simulink model "sxqq08022311"  (R2022b)
settings: Solver=VariableStepAuto  StartTime=0.0  StopTime=0.2  RelTol=1e-3
libraries: spsVoltageMeasurementLib x14, spsThyristorLib x6, spsCurrentMeasurementLib x3, spsACVoltageSourceLib x3, spsSeriesRLCBranchLib x2, spsGroundLib x1, powerlib_extras x1, spsUniversalBridgeLib x1, sps_lib x1
settings Model: Creator=赵晨琨  LastModifiedBy=ASUS
settings SolverCC: AlgebraicLoopSolver=TrustRegion
settings DataIOCC: Refine=3
settings DebuggingCC: UnconnectedInputMsg=warning  UnconnectedOutputMsg=warning  UnconnectedLineMsg=warning  SFMachineParentedDataDiag=warning
settings ModelReferenceCC: EnableRefExpFcnMdlSchedulingChecks=on

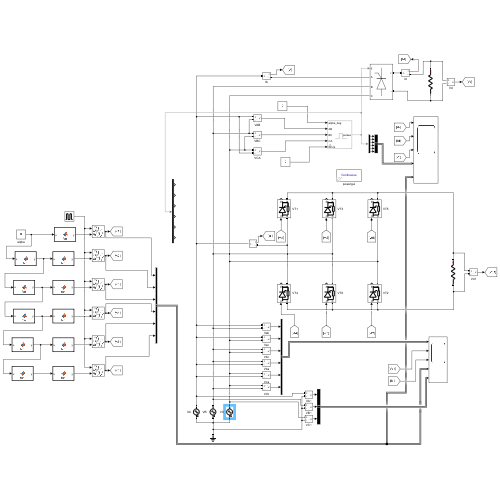
[thumbnail: Simulink's stored preview of the top-level diagram]
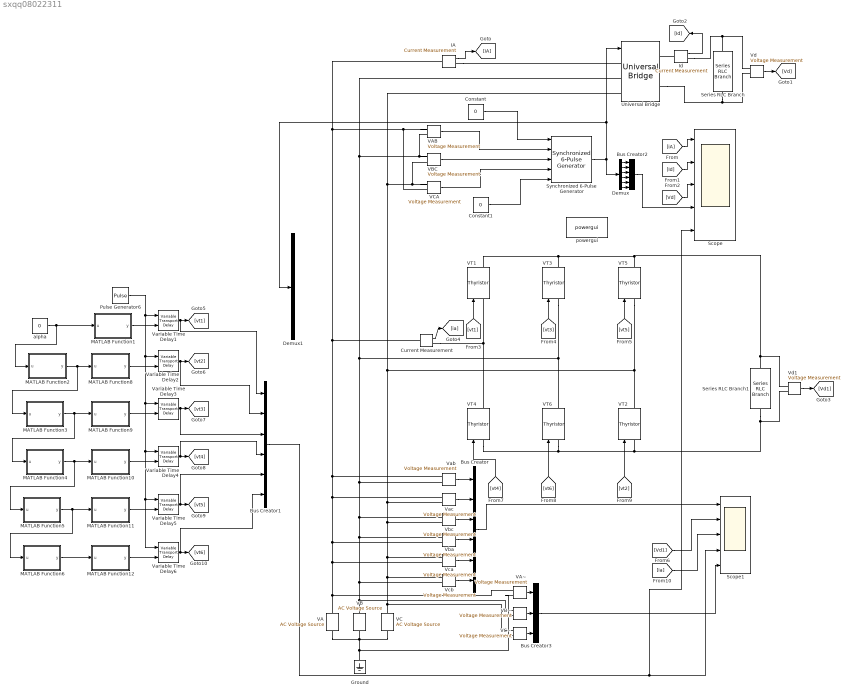
== system sxqq08022311 ==
  Bus Creator : BusCreator  Inputs=6
  Bus Creator1 : BusCreator  Inputs=6
  Bus Creator2 : BusCreator  Inputs=6
  Bus Creator3 : BusCreator  Inputs=3
  Constant : Constant  Value=0
  Constant1 : Constant  Value=0
  Current Measurement : spsCurrentMeasurementLib/Current Measurement  PhasorSimulation=off  OutputType=Complex  PSBequivalent=0
  Demux : Demux  Outputs=6
  Demux1 : Demux  Outputs=6
  Ground : spsGroundLib/Ground  LConnTagsString=a
  IA : spsCurrentMeasurementLib/Current Measurement  PhasorSimulation=off  OutputType=Complex  PSBequivalent=0
  Id : spsCurrentMeasurementLib/Current Measurement  PhasorSimulation=off  OutputType=Complex  PSBequivalent=0
  MATLAB Function1 : MATLAB Function  TreatAsAtomicUnit=on
  MATLAB Function10 : MATLAB Function  TreatAsAtomicUnit=on
  MATLAB Function11 : MATLAB Function  TreatAsAtomicUnit=on
  MATLAB Function12 : MATLAB Function  TreatAsAtomicUnit=on
  MATLAB Function2 : MATLAB Function  TreatAsAtomicUnit=on
  MATLAB Function3 : MATLAB Function  TreatAsAtomicUnit=on
  MATLAB Function4 : MATLAB Function  TreatAsAtomicUnit=on
  MATLAB Function5 : MATLAB Function  TreatAsAtomicUnit=on
  MATLAB Function6 : MATLAB Function  TreatAsAtomicUnit=on
  MATLAB Function8 : MATLAB Function  TreatAsAtomicUnit=on
  MATLAB Function9 : MATLAB Function  TreatAsAtomicUnit=on
  Pulse Generator6 : DiscretePulseGenerator  PulseType=Time based  Period=0.02  PulseWidth=20
  Scope : Scope  NumInputPorts=5
  Scope1 : Scope  NumInputPorts=5
  Series RLC Branch : spsSeriesRLCBranchLib/Series RLC Branch  LConnTagsString=__new0  RConnTagsString=__new0  BranchType=R  Resistance=1  Inductance=0  SetiL0=off  InitialCurrent=0  Capacitance=0  Setx0=off  InitialVoltage=0  Measurements=None
  Series RLC Branch1 : spsSeriesRLCBranchLib/Series RLC Branch  LConnTagsString=__new0  RConnTagsString=__new0  BranchType=R  Resistance=1  Inductance=0  SetiL0=off  InitialCurrent=0  Capacitance=0  Setx0=off  InitialVoltage=0  Measurements=None
  Synchronized 6-Pulse Generator : powerlib_extras/Control  Blocks/Synchronized 6-Pulse Generator  freq=50  pwidth=10  Double_Pulse=on
  Universal Bridge : spsUniversalBridgeLib/Universal Bridge  Arms=3  SnubberResistance=1e5  SnubberCapacitance=inf  Device=Thyristors  Ron=1e-3  Lon=0  ForwardVoltages="[  0  0  ]"  ForwardVoltage=0  GTOparameters=[ 10e-6 , 20e-6 ]  IGBTparameters=[ 1e-6 , 2e-6 ]  Measurements=None  Measurements_2=None  converterType=Rectifier
  VA : spsACVoltageSourceLib/AC Voltage Source  Amplitude=311  Phase=180  Frequency=50  SampleTime=0  Measurements=None  BusType=swing  Pref=10e3  Qref=0  Qmin=-inf  Qmax=+inf
  VAB : spsVoltageMeasurementLib/Voltage Measurement  PhasorSimulation=off  OutputType=Complex  PSBequivalent=0
  VA~ : spsVoltageMeasurementLib/Voltage Measurement  PhasorSimulation=off  OutputType=Complex  PSBequivalent=0
  "VB " : spsACVoltageSourceLib/AC Voltage Source  Amplitude=311  Phase=60  Frequency=50  SampleTime=0  Measurements=None  BusType=swing  Pref=10e3  Qref=0  Qmin=-inf  Qmax=+inf
  VBC : spsVoltageMeasurementLib/Voltage Measurement  PhasorSimulation=off  OutputType=Complex  PSBequivalent=0
  VB~ : spsVoltageMeasurementLib/Voltage Measurement  PhasorSimulation=off  OutputType=Complex  PSBequivalent=0
  VC : spsACVoltageSourceLib/AC Voltage Source  Amplitude=311  Phase=300  Frequency=50  SampleTime=0  Measurements=None  BusType=swing  Pref=10e3  Qref=0  Qmin=-inf  Qmax=+inf
  VCA : spsVoltageMeasurementLib/Voltage Measurement  PhasorSimulation=off  OutputType=Complex  PSBequivalent=0
  VC~ : spsVoltageMeasurementLib/Voltage Measurement  PhasorSimulation=off  OutputType=Complex  PSBequivalent=0
  VT{1..6} (6 alike) : spsThyristorLib/Thyristor  Ron=0.00001  Lon=0  Vf=0  IC=0  Rs=500  Cs=250e-9  Measurements=on
  Vab : spsVoltageMeasurementLib/Voltage Measurement  PhasorSimulation=off  OutputType=Complex  PSBequivalent=0
  Vac : spsVoltageMeasurementLib/Voltage Measurement  PhasorSimulation=off  OutputType=Complex  PSBequivalent=0
  Variable Time Delay{1..6} (6 alike) : VariableTransportDelay  ZeroDelay=on  TransDelayFeedthrough=on
  Vba : spsVoltageMeasurementLib/Voltage Measurement  PhasorSimulation=off  OutputType=Complex  PSBequivalent=0
  Vbc : spsVoltageMeasurementLib/Voltage Measurement  PhasorSimulation=off  OutputType=Complex  PSBequivalent=0
  Vca : spsVoltageMeasurementLib/Voltage Measurement  PhasorSimulation=off  OutputType=Complex  PSBequivalent=0
  Vcb : spsVoltageMeasurementLib/Voltage Measurement  PhasorSimulation=off  OutputType=Complex  PSBequivalent=0
  Vd : spsVoltageMeasurementLib/Voltage Measurement  PhasorSimulation=off  OutputType=Complex  PSBequivalent=0
  Vd1 : spsVoltageMeasurementLib/Voltage Measurement  PhasorSimulation=off  OutputType=Complex  PSBequivalent=0
  alpha : Constant  Value=0
  powergui : sps_lib/powergui  Priority=1  SimulationMode=Continuous  SampleTime=5e-5  frequency=60  Iterations=50  frequencyindice=50  Pbase=100e6  ErrMax=1e-4  UnitsV=kV  UnitsW=MW  buscounter=0  FunctionMessages=off  echomessages=off  EnableUseOfTLC=off  CurrentSourceSwitches=off  DisableSnubberDevices=off  DisableRonSwitches=off  DisableVfSwitches=off  DisplayEquations=off  AutomaticDiscreteSolvers=off  SolverType=Tustin/Backward Euler (TBE)  Interpol=off  ExternalGateDelay=off  methode=off  Ts=100  x0status=blocks  SPID=on  SwTol=0  HookPort=off  NonlinearTolerance=1e-4  nMaxIteration=100  ContinueOnMaxIteration=off  RestoreLinks=warning  ResistiveCurrentMeasurement=off  Frange=[0:2:500]  Ylog=off  Xlog=on  ShowGrid=off  save=off  variable=ZData  structure=0  ZoomFFT=off  StartTime=0.0  cycles=1  DisplayStyle=1  fundamental=60  FreqAxis=off  MaxFrequency=1000  frequencyindicesteady=1  RmsSteady=1  display=off
  wires:
  Constant1/1 -> Synchronized 6-Pulse Generator/5
  Constant/1 -> Synchronized 6-Pulse Generator/1
  VAB/1 -> Synchronized 6-Pulse Generator/2
  VBC/1 -> Synchronized 6-Pulse Generator/3
  VCA/1 -> Synchronized 6-Pulse Generator/4
  Synchronized 6-Pulse Generator/1 -> Demux1/1, Universal Bridge/1, Demux/1
  IA/1 -> [iA]
  Vd/1 -> [Vd]
  Id/1 -> [Id]
  [iA] -> Scope/1
  [Id] -> Scope/2
  [Vd] -> Scope/3
  Vd1/1 -> [Vd1]
  Vab/1 -> Bus Creator/1
  Vac/1 -> Bus Creator/2
  Vba/1 -> Bus Creator/4
  Vca/1 -> Bus Creator/5
  Vcb/1 -> Bus Creator/6
  Vbc/1 -> Bus Creator/3
  Bus Creator/1 -> Scope1/1
  MATLAB Function1/1(y) -> Variable Time Delay1/2
  alpha/1 -> MATLAB Function2/1(u), MATLAB Function1/1(u)
  MATLAB Function2/1(y) -> MATLAB Function3/1(u), MATLAB Function8/1(u)
  MATLAB Function3/1(y) -> MATLAB Function9/1(u), MATLAB Function4/1(u)
  MATLAB Function4/1(y) -> MATLAB Function10/1(u), MATLAB Function5/1(u)
  MATLAB Function5/1(y) -> MATLAB Function11/1(u), MATLAB Function6/1(u)
  MATLAB Function6/1(y) -> MATLAB Function12/1(u)
  MATLAB Function8/1(y) -> Variable Time Delay2/2
  MATLAB Function9/1(y) -> Variable Time Delay3/2
  MATLAB Function10/1(y) -> Variable Time Delay4/2
  MATLAB Function11/1(y) -> Variable Time Delay5/2
  MATLAB Function12/1(y) -> Variable Time Delay6/2
  Pulse Generator6/1 -> Variable Time Delay6/1, Variable Time Delay5/1, Variable Time Delay4/1, Variable Time Delay3/1, Variable Time Delay2/1, Variable Time Delay1/1
  Variable Time Delay1/1 -> Bus Creator1/1, [vt1]
  Variable Time Delay2/1 -> Bus Creator1/2, [vt2]
  Variable Time Delay3/1 -> Bus Creator1/3, [vt3]
  Variable Time Delay6/1 -> Bus Creator1/6, [vt6]
  Variable Time Delay4/1 -> Bus Creator1/4, [vt4]
  Variable Time Delay5/1 -> Bus Creator1/5, [vt5]
  [Vd1] -> Scope1/2
  [ia] -> Scope1/3
  Bus Creator1/1 -> Scope/5, Scope1/4
  Demux/1 -> Bus Creator2/1
  Bus Creator2/1 -> Scope/4
  Current Measurement/1 -> [ia]
  Demux/6 -> Bus Creator2/6
  Demux/2 -> Bus Creator2/2
  Demux/3 -> Bus Creator2/3
  Demux/4 -> Bus Creator2/4
  Demux/5 -> Bus Creator2/5
  [vt1] -> VT1/1
  [vt3] -> VT3/1
  [vt5] -> VT5/1
  [vt4] -> VT4/1
  [vt6] -> VT6/1
  [vt2] -> VT2/1
  VA~/1 -> Bus Creator3/1
  VB~/1 -> Bus Creator3/2
  VC~/1 -> Bus Creator3/3
  Bus Creator3/1 -> Scope1/5
  connections:
  Series RLC Branch/LConn1 -- Id/RConn1 -- Vd/LConn1
  Universal Bridge/RConn2 -- Series RLC Branch/RConn1 -- Vd/LConn2
  VA/RConn1 -- VC/RConn1 -- "VB "/RConn1 -- VB~/LConn2 -- VA~/LConn2 -- VC~/LConn2 -- Ground/LConn1
  VA/LConn1 -- VA~/LConn1 -- Vca/LConn2 -- Vba/LConn2 -- Vab/LConn1 -- Current Measurement/LConn1 -- IA/LConn1 -- VAB/LConn1 -- VCA/LConn2 -- Vac/LConn1
  "VB "/LConn1 -- Vcb/LConn2 -- Vba/LConn1 -- Vbc/LConn1 -- Vab/LConn2 -- VT6/RConn1 -- VT3/LConn1 -- VAB/LConn2 -- VBC/LConn1 -- Universal Bridge/LConn2 -- VB~/LConn1
  VC/LConn1 -- Vcb/LConn1 -- Vca/LConn1 -- Vbc/LConn2 -- Vac/LConn2 -- VT5/LConn1 -- VT2/RConn1 -- VCA/LConn1 -- VBC/LConn2 -- Universal Bridge/LConn3 -- VC~/LConn1
  IA/RConn1 -- Universal Bridge/LConn1
  Id/LConn1 -- Universal Bridge/RConn1
  Series RLC Branch1/LConn1 -- VT1/RConn1 -- VT3/RConn1 -- VT5/RConn1 -- Vd1/LConn1
  VT6/LConn1 -- VT4/LConn1 -- Series RLC Branch1/RConn1 -- Vd1/LConn2 -- VT2/LConn1
  VT4/RConn1 -- Current Measurement/RConn1 -- VT1/LConn1

== matlab function sxqq08022311/MATLAB Function2 ==
  data: u input; y output
function y = fcn(u)
y = u+60;

== matlab function sxqq08022311/MATLAB Function3 ==
  data: u input; y output
function y = fcn(u)

y = u+60;

== matlab function sxqq08022311/MATLAB Function4 ==
  data: u input; y output
function y = fcn(u)

y = u+60;

== matlab function sxqq08022311/MATLAB Function5 ==
  data: u input; y output
function y = fcn(u)

y = u+60;

== matlab function sxqq08022311/MATLAB Function6 ==
  data: u input; y output
function y = fcn(u)

y = u+60;

== matlab function sxqq08022311/MATLAB Function8 ==
  data: u input; y output
function y = fcn(u)
y = (u+30)/360/50;

== matlab function sxqq08022311/MATLAB Function9 ==
  data: u input; y output
function y = fcn(u)

y = (u+30)/360/50;

== matlab function sxqq08022311/MATLAB Function10 ==
  data: u input; y output
function y = fcn(u)

y = (u+30)/360/50;

== matlab function sxqq08022311/MATLAB Function1 ==
  data: u input; y output
function y = fcn(u)

y = (u+30)/360/50;

== matlab function sxqq08022311/MATLAB Function11 ==
  data: u input; y output
function y = fcn(u)

y = (u+30)/360/50;

== matlab function sxqq08022311/MATLAB Function12 ==
  data: u input; y output
function y = fcn(u)

y = (u+30)/360/50;
